simulink model "LAB_Stima_e_Controllo_Lez_7_Filtro_di_Kalman_Simulink"  (R2018a)
settings: Solver=VariableStepAuto  StartTime=0.0  StopTime=100.0  RelTol=1e-3
values from neighbouring files (symbols this model uses):
  A = [0 1 0;0 -f/J km/J;0 -kv/La -Ra/La]    [LAB_Stima_e_Controllo_Lez_1_Motore_Corrente_Continua.m]    (also in LAB_Stima_e_Controllo_Lez_2_Sistema_Idraulico.m = [-a a 0;a -2*a a;0 a -(a+b)]; LAB_Stima_e_Controllo_Lez_4_Pendolo_Inverso.m = [0 1 0 0;0 0 -(m*g)/M 0;0 0 0 1;0 0 ((M+m)*g)/(M*L) 0]; LAB_Stima_e_Controllo_Lez_6_Filtro_di_Kalman_TC.m; LAB_Stima_e_Controllo_Lez_6_Filtro_di_Kalman_TD.m = [1.1269 -0.4940 0.1129;1 0 0;0 1 0])
  B = [0;0;Ga/La]    [LAB_Stima_e_Controllo_Lez_1_Motore_Corrente_Continua.m]    (also in LAB_Stima_e_Controllo_Lez_2_Sistema_Idraulico.m = [1/S 0;0 0;0 1/S]; LAB_Stima_e_Controllo_Lez_4_Pendolo_Inverso.m = [0;1/M;0;-1/(M*L)]; LAB_Stima_e_Controllo_Lez_6_Filtro_di_Kalman_TC.m; LAB_Stima_e_Controllo_Lez_6_Filtro_di_Kalman_TD.m = [-0.3832;0.5919;0.5191])
  C = [1 0 0]    [LAB_Stima_e_Controllo_Lez_1_Motore_Corrente_Continua.m]    (also in LAB_Stima_e_Controllo_Lez_2_Sistema_Idraulico.m = [0 0 1]; LAB_Stima_e_Controllo_Lez_4_Pendolo_Inverso.m = [1 0 0 0;0 0 1 0]; LAB_Stima_e_Controllo_Lez_6_Filtro_di_Kalman_TC.m; LAB_Stima_e_Controllo_Lez_6_Filtro_di_Kalman_TD.m)
  D = 0    [LAB_Stima_e_Controllo_Lez_1_Motore_Corrente_Continua.m]    (also in LAB_Stima_e_Controllo_Lez_2_Sistema_Idraulico.m = [0 0]; LAB_Stima_e_Controllo_Lez_4_Pendolo_Inverso.m; LAB_Stima_e_Controllo_Lez_6_Filtro_di_Kalman_TC.m; LAB_Stima_e_Controllo_Lez_6_Filtro_di_Kalman_TD.m)
undefined symbols (not defined in the file or in its folder): Continuous, Time
libraries: ctrlSharedLib x1
settings Model: Creator=anton  LastModifiedBy=anton

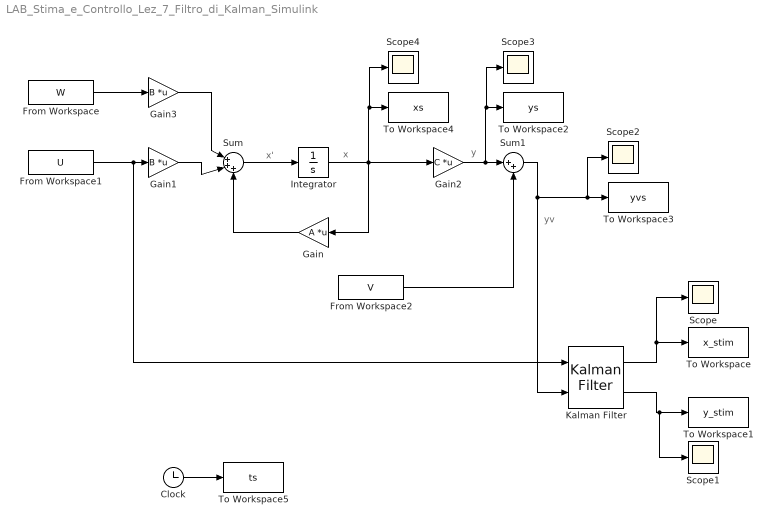
== system LAB_Stima_e_Controllo_Lez_7_Filtro_di_Kalman_Simulink ==
  note: yv
  note: y
  note: x
  note: x'
  Clock : Clock
  From Workspace : FromWorkspace  VariableName=W  SampleTime=0
  From Workspace1 : FromWorkspace  VariableName=U  SampleTime=0
  From Workspace2 : FromWorkspace  VariableName=V  SampleTime=0
  Gain : Gain  Gain=A  Multiplication=Matrix(K*u)
  Gain1 : Gain  Gain=B  Multiplication=Matrix(K*u)
  Gain2 : Gain  Gain=C  Multiplication=Matrix(K*u)
  Gain3 : Gain  Gain=B  Multiplication=Matrix(K*u)
  Integrator : Integrator
  Kalman Filter : ctrlSharedLib/Kalman Filter  TimeDomain=Continuous-Time  UseCurrentEstimator=on  ModelSource=LTI State-Space Variable  ModelSourceVariable=ss(A,B,C,D)  A=0.95  B=1  C=1  D=0  NumberOfStates=1  NumberOfInputs=1  NumberOfOutputs=1  InitialEstimateSource=Dialog  X0=0  P0=10  UseK=off  UseGH=off  NumberOfProcessNoiseInputs=1  G=1  TimeInvariantG=on  H=0  TimeInvariantH=on  Q=1  TimeInvariantQ=on  R=1  TimeInvariantR=on  N=0  TimeInvariantN=on  AddInputPort=on  AddEnablePort=off  OutputEstimatedY=on  OutputP=off  Ts=-1
      settings: SourceProductBaseCode=CT
  Scope{,1..4} (5 alike) : Scope
  Sum : Sum  Inputs=|+++
  Sum1 : Sum  Inputs=|++
  To Workspace : ToWorkspace  VariableName=x_stim  SampleTime=-1
  To Workspace1 : ToWorkspace  VariableName=y_stim  SampleTime=-1
  To Workspace2 : ToWorkspace  VariableName=ys  SampleTime=-1
  To Workspace3 : ToWorkspace  VariableName=yvs  SampleTime=-1
  To Workspace4 : ToWorkspace  VariableName=xs  SampleTime=-1
  To Workspace5 : ToWorkspace  VariableName=ts  SampleTime=-1
  wires:
  Integrator/1 -> Scope4/1, To Workspace4/1, Gain/1, Gain2/1
  Sum/1 -> Integrator/1
  Gain/1 -> Sum/3
  Gain1/1 -> Sum/2
  Gain3/1 -> Sum/1
  From Workspace/1 -> Gain3/1
  From Workspace1/1 -> Kalman Filter/1, Gain1/1
  Gain2/1 -> Scope3/1, To Workspace2/1, Sum1/1
  From Workspace2/1 -> Sum1/2
  Sum1/1 -> Scope2/1, To Workspace3/1, Kalman Filter/2
  Kalman Filter/1 -> Scope/1, To Workspace/1
  Kalman Filter/2 -> Scope1/1, To Workspace1/1
  Clock/1 -> To Workspace5/1
